simulink model "Control_simulacion_obsv_miercoles"  (R2016a)
settings: Solver=VariableStepAuto  StartTime=0.0  StopTime=60  RelTol=1e-3
values from neighbouring files (symbols this model uses):
  Ac_2 = [ALn-BLn*Kest-L*CLn+L*DLn*Kest, BLn*Ki - L*DLn*Ki ... (first row only)    [Control_MIMO_Observador_continua.m]
  ALn = double(subs(AL,{a,b,c,d},{a1,b1,c1,d1}))    [Control_MIMO_Observador_continua.m]
  Bc_2 = [zeros(n,r),L ... (first row only)    [Control_MIMO_Observador_continua.m]
  BLn = double(subs(BL,{a,b,c,d},{a1,b1,c1,d1}))    [Control_MIMO_Observador_continua.m]
  Cc_2 = [-Kest, Ki]    [Control_MIMO_Observador_continua.m]
  CLn = [1 0 0 ... (first row only)    [Control_MIMO_Observador_continua.m]
  Dc_2 = zeros(p,2*r)    [Control_MIMO_Observador_continua.m]
  DLn = [0 0 0 ... (first row only)    [Control_MIMO_Observador_continua.m]
  Kest = K(:,1:n)    [Control_MIMO_Observador_continua.m]
  Ki = -K(:,n+1:end)    [Control_MIMO_Observador_continua.m]
  L = (Grand*inv(X))'    [Control_MIMO_Observador_continua.m]
  u10 = double((a1*x20 + b1*x10^2)/u20)    [Control_MIMO_Observador_continua.m]
  u20 = double(sqrt(c1*x30*x20))    [Control_MIMO_Observador_continua.m]
  u30 = double((d1*x30 - u10)/x10)    [Control_MIMO_Observador_continua.m]
  x10 = 2    [Control_MIMO_Observador_continua.m]
  x20 = 4    [Control_MIMO_Observador_continua.m]
  x30 = 4    [Control_MIMO_Observador_continua.m]
libraries: cstblocks x1
settings Model: Creator=Lenovo  LastModifiedBy=Lenovo

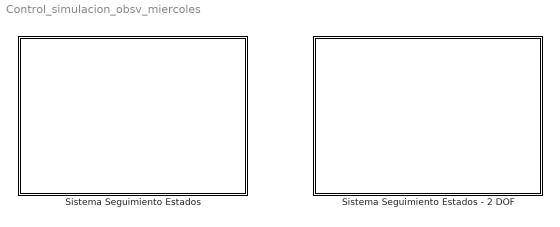
== system Control_simulacion_obsv_miercoles ==
  Sistema Seguimiento Estados : Subsystem
  Sistema Seguimiento Estados - 2 DOF : Subsystem

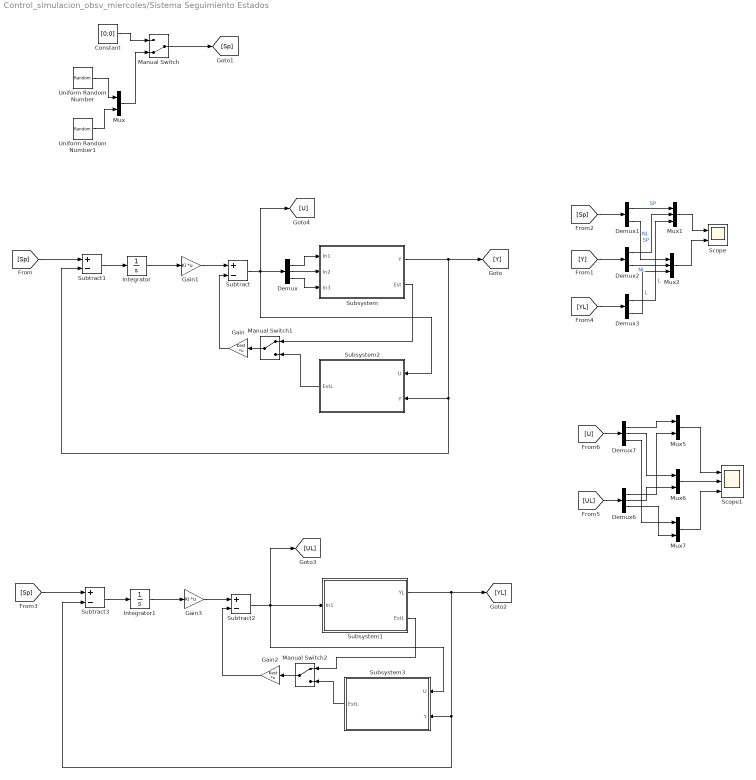
== system Control_simulacion_obsv_miercoles/Sistema Seguimiento Estados ==
  Constant : Constant  Value=[0;0]
  Demux : Demux  Outputs=3
  Demux1 : Demux  Outputs=2
  Demux2 : Demux  Outputs=2
  Demux3 : Demux  Outputs=2
  Demux6 : Demux  Outputs=3
  Demux7 : Demux  Outputs=3
  Gain : Gain  Gain=Kest  Multiplication=Matrix(K*u)
  Gain1 : Gain  Gain=Ki  Multiplication=Matrix(K*u)
  Gain2 : Gain  Gain=Kest  Multiplication=Matrix(K*u)
  Gain3 : Gain  Gain=Ki  Multiplication=Matrix(K*u)
  Integrator : Integrator
  Integrator1 : Integrator
  Manual Switch : ManualSwitch  CurrentSetting=0
  Manual Switch1 : ManualSwitch
  Manual Switch2 : ManualSwitch
  Mux{,5..7} (4 alike) : Mux  Inputs=2
  Mux1 : Mux  Inputs=3
  Mux2 : Mux  Inputs=3
  Scope : Scope  NumInputPorts=2
  Scope1 : Scope  NumInputPorts=3
  Subsystem : Subsystem
  Subsystem1 : Subsystem
  Subsystem2 : Subsystem
  Subsystem3 : Subsystem
  Subtract{,1..3} (4 alike) : Sum  Inputs=+-
  Uniform Random Number : UniformRandomNumber  Minimum=-0.2  Maximum=0.2  SampleTime=3
  Uniform Random Number1 : UniformRandomNumber  Minimum=-0.4  Maximum=0.4  SampleTime=7
  wires:
  Constant/1 -> Manual Switch/1
  Mux/1 -> Manual Switch/2
  Manual Switch/1 -> [Sp]
  Demux1/2 -> Mux2/1  "SP"
  [Sp] -> Demux1/1
  [Y] -> Demux2/1
  Demux2/1 -> Mux1/2  "NL"
  Demux1/1 -> Mux1/1  "SP"
  Demux2/2 -> Mux2/2  "NL"
  Uniform Random Number1/1 -> Mux/2
  Uniform Random Number/1 -> Mux/1
  Demux/3 -> Subsystem/3(In3)
  Demux/2 -> Subsystem/2(In2)
  Demux/1 -> Subsystem/1(In1)
  Subtract/1 -> Subsystem2/1(U), [U], Demux/1
  Demux3/1 -> Mux1/3  "L"
  Subsystem1/1(YL) -> Subsystem3/2(Y), Subtract3/2, [YL]
  Gain3/1 -> Subtract2/1
  Gain2/1 -> Subtract2/2
  [Sp] -> Subtract3/1
  [YL] -> Demux3/1
  Subtract2/1 -> Subsystem3/1(U), [UL], Subsystem1/1(In1)
  Demux3/2 -> Mux2/3  "L"
  Subsystem/1(Y) -> Subsystem2/2(Y), Subtract1/2, [Y]
  Mux2/1 -> Scope/2
  Mux1/1 -> Scope/1
  Gain/1 -> Subtract/2
  Gain1/1 -> Subtract/1
  [Sp] -> Subtract1/1
  [UL] -> Demux6/1
  [U] -> Demux7/1
  Demux7/1 -> Mux5/1
  Demux6/1 -> Mux5/2
  Demux7/2 -> Mux6/1
  Demux6/2 -> Mux6/2
  Demux7/3 -> Mux7/1
  Demux6/3 -> Mux7/2
  Mux5/1 -> Scope1/1
  Mux6/1 -> Scope1/2
  Mux7/1 -> Scope1/3
  Integrator/1 -> Gain1/1
  Subtract1/1 -> Integrator/1
  Integrator1/1 -> Gain3/1
  Subtract3/1 -> Integrator1/1
  Manual Switch1/1 -> Gain/1
  Subsystem/2(Est) -> Manual Switch1/1
  Subsystem2/1(EstL) -> Manual Switch1/2
  Manual Switch2/1 -> Gain2/1
  Subsystem3/1(EstL) -> Manual Switch2/2
  Subsystem1/2(EstL) -> Manual Switch2/1

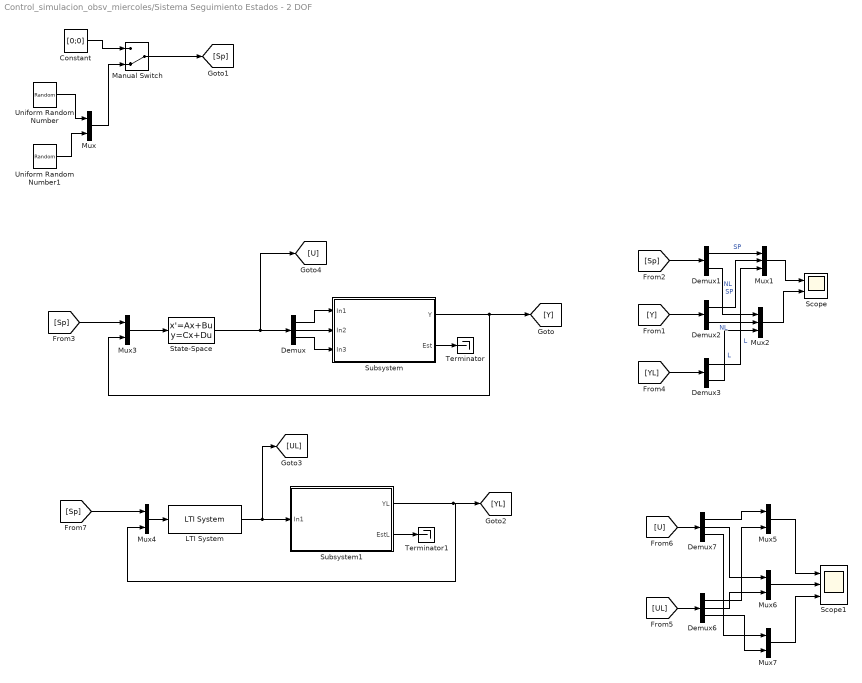
== system Control_simulacion_obsv_miercoles/Sistema Seguimiento Estados - 2 DOF ==
  Constant : Constant  Value=[0;0]
  Demux : Demux  Outputs=3
  Demux1 : Demux  Outputs=2
  Demux2 : Demux  Outputs=2
  Demux3 : Demux  Outputs=2
  Demux6 : Demux  Outputs=3
  Demux7 : Demux  Outputs=3
  LTI System : cstblocks/LTI System  sys=sys_c2  IC=[]
  Manual Switch : ManualSwitch  CurrentSetting=0
  Mux{,3..7} (6 alike) : Mux  Inputs=2
  Mux1 : Mux  Inputs=3
  Mux2 : Mux  Inputs=3
  Scope : Scope  NumInputPorts=2
  Scope1 : Scope  NumInputPorts=3
  State-Space : StateSpace  A=Ac_2  B=Bc_2  C=Cc_2  D=Dc_2  X0=0
  Subsystem : Subsystem
  Subsystem1 : Subsystem
  Terminator : Terminator
  Terminator1 : Terminator
  Uniform Random Number : UniformRandomNumber  Minimum=-0.2  Maximum=0.2  SampleTime=3
  Uniform Random Number1 : UniformRandomNumber  Minimum=-0.4  Maximum=0.4  SampleTime=7
  wires:
  Constant/1 -> Manual Switch/1
  Mux/1 -> Manual Switch/2
  Manual Switch/1 -> [Sp]
  Demux1/2 -> Mux2/1  "SP"
  [Sp] -> Demux1/1
  [Y] -> Demux2/1
  Demux2/1 -> Mux1/2  "NL"
  Demux1/1 -> Mux1/1  "SP"
  Demux2/2 -> Mux2/2  "NL"
  Uniform Random Number1/1 -> Mux/2
  Uniform Random Number/1 -> Mux/1
  Demux/3 -> Subsystem/3(In3)
  Demux/2 -> Subsystem/2(In2)
  Demux/1 -> Subsystem/1(In1)
  State-Space/1 -> [U], Demux/1
  Demux3/1 -> Mux1/3  "L"
  Subsystem1/1(YL) -> Mux4/2, [YL]
  [YL] -> Demux3/1
  Demux3/2 -> Mux2/3  "L"
  Subsystem/1(Y) -> Mux3/2, [Y]
  Mux2/1 -> Scope/2
  Mux1/1 -> Scope/1
  [UL] -> Demux6/1
  [U] -> Demux7/1
  Demux7/1 -> Mux5/1
  Demux6/1 -> Mux5/2
  Demux7/2 -> Mux6/1
  Demux6/2 -> Mux6/2
  Demux7/3 -> Mux7/1
  Demux6/3 -> Mux7/2
  Mux5/1 -> Scope1/1
  Mux6/1 -> Scope1/2
  Mux7/1 -> Scope1/3
  Mux3/1 -> State-Space/1
  [Sp] -> Mux3/1
  Subsystem/2(Est) -> Terminator/1
  [Sp] -> Mux4/1
  LTI System/1 -> [UL], Subsystem1/1(In1)
  Mux4/1 -> LTI System/1
  Subsystem1/2(EstL) -> Terminator1/1

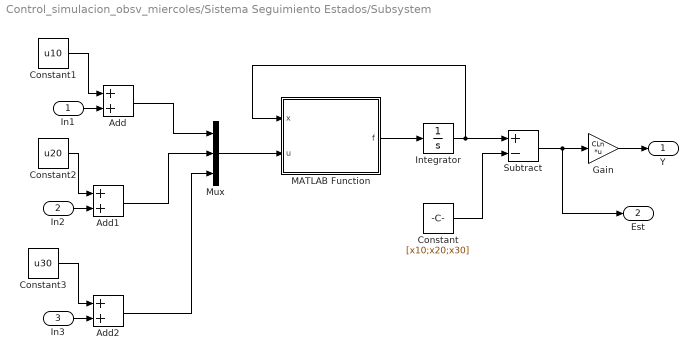
== system Control_simulacion_obsv_miercoles/Sistema Seguimiento Estados/Subsystem ==
  In1 : Inport
  In2 : Inport  Port=2
  In3 : Inport  Port=3
  Add : Sum
  Add1 : Sum
  Add2 : Sum
  Constant : Constant  Value=[x10;x20;x30]
  Constant1 : Constant  Value=u10
  Constant2 : Constant  Value=u20
  Constant3 : Constant  Value=u30
  Gain : Gain  Gain=CLn  Multiplication=Matrix(K*u)
  Integrator : Integrator  InitialCondition=[x10;x20;x30]
  MATLAB Function : MATLAB Function  TreatAsAtomicUnit=on
  Mux : Mux  Inputs=3
  Subtract : Sum  Inputs=+-
  Y : Outport
  Est : Outport  Port=2
  wires:
  Add2/1 -> Mux/3
  Mux/1 -> MATLAB Function/2(u)
  Constant2/1 -> Add1/1
  Constant1/1 -> Add/1
  Constant3/1 -> Add2/1
  Integrator/1 -> MATLAB Function/1(x), Subtract/1
  Add/1 -> Mux/1
  Add1/1 -> Mux/2
  In2/1 -> Add1/2
  Gain/1 -> Y/1
  In1/1 -> Add/2
  In3/1 -> Add2/2
  MATLAB Function/1(f) -> Integrator/1
  Subtract/1 -> Est/1, Gain/1
  Constant/1 -> Subtract/2

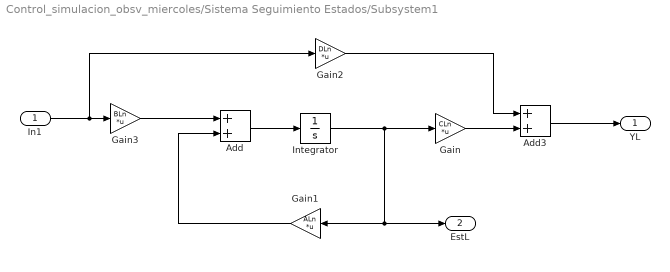
== system Control_simulacion_obsv_miercoles/Sistema Seguimiento Estados/Subsystem1 ==
  In1 : Inport
  Add : Sum
  Add3 : Sum
  Gain : Gain  Gain=CLn  Multiplication=Matrix(K*u)
  Gain1 : Gain  Gain=ALn  Multiplication=Matrix(K*u)
  Gain2 : Gain  Gain=DLn  Multiplication=Matrix(K*u)
  Gain3 : Gain  Gain=BLn  Multiplication=Matrix(K*u)
  Integrator : Integrator
  YL : Outport
  EstL : Outport  Port=2
  wires:
  Add/1 -> Integrator/1
  Gain1/1 -> Add/2
  Integrator/1 -> Gain/1, EstL/1, Gain1/1
  Gain/1 -> Add3/2
  Add3/1 -> YL/1
  Gain2/1 -> Add3/1
  Gain3/1 -> Add/1
  In1/1 -> Gain2/1, Gain3/1

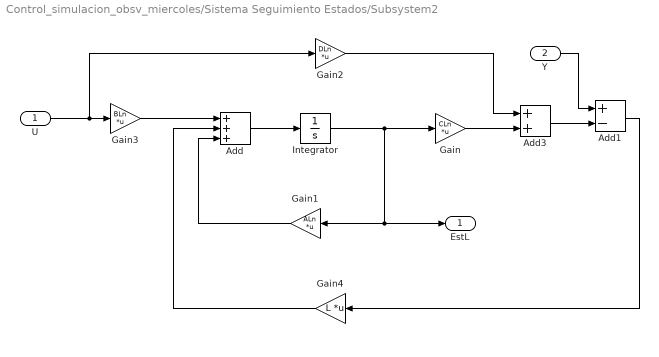
== system Control_simulacion_obsv_miercoles/Sistema Seguimiento Estados/Subsystem2 ==
  U : Inport
  Y : Inport  Port=2
  Add : Sum  Inputs=+++
  Add1 : Sum  Inputs=+-
  Add3 : Sum
  Gain : Gain  Gain=CLn  Multiplication=Matrix(K*u)
  Gain1 : Gain  Gain=ALn  Multiplication=Matrix(K*u)
  Gain2 : Gain  Gain=DLn  Multiplication=Matrix(K*u)
  Gain3 : Gain  Gain=BLn  Multiplication=Matrix(K*u)
  Gain4 : Gain  Gain=L  Multiplication=Matrix(K*u)
  Integrator : Integrator
  EstL : Outport
  wires:
  Add/1 -> Integrator/1
  Integrator/1 -> Gain/1, EstL/1, Gain1/1
  Gain/1 -> Add3/2
  Gain2/1 -> Add3/1
  Gain3/1 -> Add/1
  U/1 -> Gain2/1, Gain3/1
  Add3/1 -> Add1/2
  Y/1 -> Add1/1
  Add1/1 -> Gain4/1
  Gain1/1 -> Add/3
  Gain4/1 -> Add/2

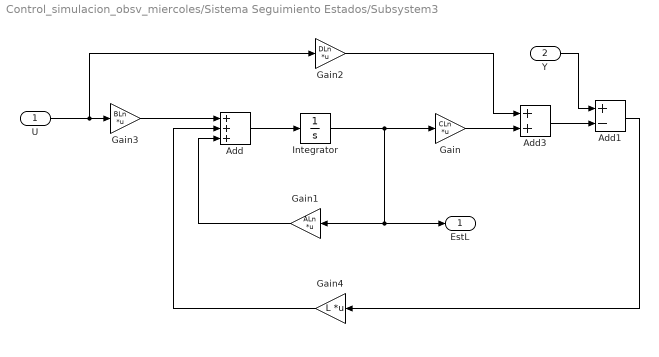
== system Control_simulacion_obsv_miercoles/Sistema Seguimiento Estados/Subsystem3 ==
  U : Inport
  Y : Inport  Port=2
  Add : Sum  Inputs=+++
  Add1 : Sum  Inputs=+-
  Add3 : Sum
  Gain : Gain  Gain=CLn  Multiplication=Matrix(K*u)
  Gain1 : Gain  Gain=ALn  Multiplication=Matrix(K*u)
  Gain2 : Gain  Gain=DLn  Multiplication=Matrix(K*u)
  Gain3 : Gain  Gain=BLn  Multiplication=Matrix(K*u)
  Gain4 : Gain  Gain=L  Multiplication=Matrix(K*u)
  Integrator : Integrator
  EstL : Outport
  wires:
  Add/1 -> Integrator/1
  Integrator/1 -> Gain/1, EstL/1, Gain1/1
  Gain/1 -> Add3/2
  Gain2/1 -> Add3/1
  Gain3/1 -> Add/1
  U/1 -> Gain2/1, Gain3/1
  Add3/1 -> Add1/2
  Y/1 -> Add1/1
  Add1/1 -> Gain4/1
  Gain1/1 -> Add/3
  Gain4/1 -> Add/2

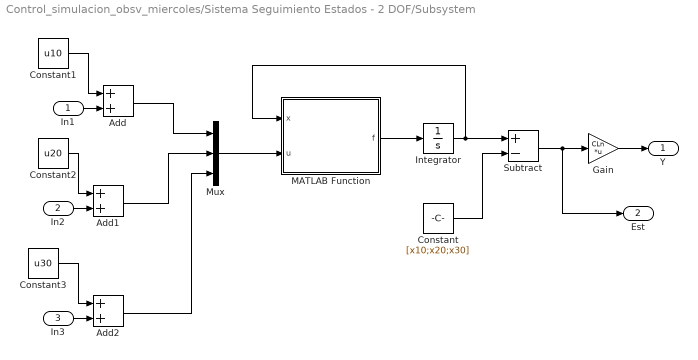
== system Control_simulacion_obsv_miercoles/Sistema Seguimiento Estados - 2 DOF/Subsystem ==
  In1 : Inport
  In2 : Inport  Port=2
  In3 : Inport  Port=3
  Add : Sum
  Add1 : Sum
  Add2 : Sum
  Constant : Constant  Value=[x10;x20;x30]
  Constant1 : Constant  Value=u10
  Constant2 : Constant  Value=u20
  Constant3 : Constant  Value=u30
  Gain : Gain  Gain=CLn  Multiplication=Matrix(K*u)
  Integrator : Integrator  InitialCondition=[x10;x20;x30]
  MATLAB Function : MATLAB Function  TreatAsAtomicUnit=on
  Mux : Mux  Inputs=3
  Subtract : Sum  Inputs=+-
  Y : Outport
  Est : Outport  Port=2
  wires:
  Add2/1 -> Mux/3
  Mux/1 -> MATLAB Function/2(u)
  Constant2/1 -> Add1/1
  Constant1/1 -> Add/1
  Constant3/1 -> Add2/1
  Integrator/1 -> MATLAB Function/1(x), Subtract/1
  Add/1 -> Mux/1
  Add1/1 -> Mux/2
  In2/1 -> Add1/2
  Gain/1 -> Y/1
  In1/1 -> Add/2
  In3/1 -> Add2/2
  MATLAB Function/1(f) -> Integrator/1
  Subtract/1 -> Est/1, Gain/1
  Constant/1 -> Subtract/2

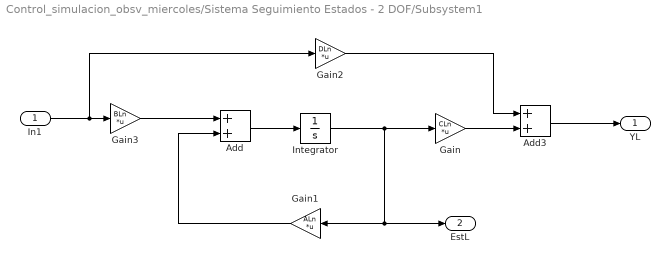
== system Control_simulacion_obsv_miercoles/Sistema Seguimiento Estados - 2 DOF/Subsystem1 ==
  In1 : Inport
  Add : Sum
  Add3 : Sum
  Gain : Gain  Gain=CLn  Multiplication=Matrix(K*u)
  Gain1 : Gain  Gain=ALn  Multiplication=Matrix(K*u)
  Gain2 : Gain  Gain=DLn  Multiplication=Matrix(K*u)
  Gain3 : Gain  Gain=BLn  Multiplication=Matrix(K*u)
  Integrator : Integrator
  YL : Outport
  EstL : Outport  Port=2
  wires:
  Add/1 -> Integrator/1
  Gain1/1 -> Add/2
  Integrator/1 -> Gain/1, EstL/1, Gain1/1
  Gain/1 -> Add3/2
  Add3/1 -> YL/1
  Gain2/1 -> Add3/1
  Gain3/1 -> Add/1
  In1/1 -> Gain2/1, Gain3/1

== matlab function Control_simulacion_obsv_miercoles/Sistema Seguimiento Estados - 2 DOF/Subsystem/MATLAB Function ==
  data: x input; u input; f output
function f = fcn(x,u)

a = 2;
b = 4;
c = 1;
d = 3;

x1 = x(1);
x2 = x(2);
x3 = x(3);
u1 = u(1);
u2 = u(2);
u3 = u(3);
f1 = -a*x2 - b*x1^2 + u1*u2;
f2 = -c*x3*x2 + u2^2 ;
f3 = -d*x3 + u3*x1 + u1;
f = [f1; f2; f3];

== matlab function Control_simulacion_obsv_miercoles/Sistema Seguimiento Estados/Subsystem/MATLAB Function ==
  data: x input; u input; f output
function f = fcn(x,u)

a = 2;
b = 4;
c = 1;
d = 3;

x1 = x(1);
x2 = x(2);
x3 = x(3);
u1 = u(1);
u2 = u(2);
u3 = u(3);
f1 = -a*x2 - b*x1^2 + u1*u2;
f2 = -c*x3*x2 + u2^2 ;
f3 = -d*x3 + u3*x1 + u1;
f = [f1; f2; f3];
